simulink model "HIL"  (R2023b)
settings: Solver=VariableStepAuto  StartTime=0.0  StopTime=20.0  RelTol=1e-3
model workspace (MAT data in the model file):
  Iq_ref : Simulink.Parameter (value not decoded)
  Ki_d : Simulink.Parameter (value not decoded)
  Ki_q : Simulink.Parameter (value not decoded)
  Kp_d : Simulink.Parameter (value not decoded)
  Kp_q : Simulink.Parameter (value not decoded)
  P : Simulink.Parameter (value not decoded)
  Torq : Simulink.Parameter (value not decoded)
  Vdc : Simulink.Parameter (value not decoded)
  fe : Simulink.Parameter (value not decoded)
symbols that are objects in the model workspace (value not decoded): fe, Ki_d, Kp_d, P, Torq, Vdc
libraries: instrumentseriallib x3, etargetslib x2, slpidlib x2, mcbcontrolslib x1, dspfdesign x1, dspstat3 x1
(part 2 of 2)

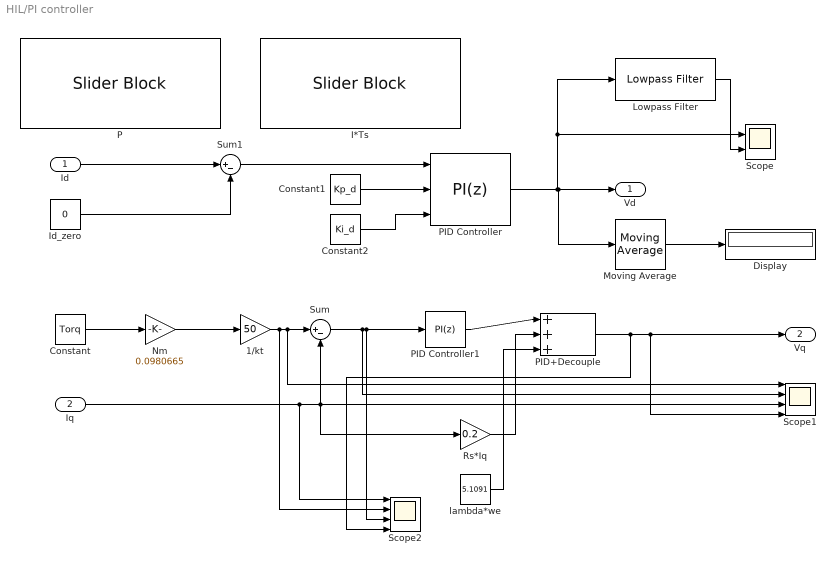
== system HIL/PI controller ==
  Id : Inport
  Iq : Inport  Port=2
  1/kt : Gain  Gain=50
  Constant : Constant  Value=Torq
  Constant1 : Constant  Value=Kp_d
  Constant2 : Constant  Value=Ki_d
  Display : Display
  I*Ts : SliderBlock  ScaleMax=0.1
  Id_zero : Constant  Value=0
  Lowpass Filter : dspfdesign/Lowpass Filter  FilterType=FIR  DesignForMinimumOrder=on  FilterOrder=50  PassbandFrequency=8e3  StopbandFrequency=12e3  PassbandRipple=0.1  StopbandAttenuation=80  SampleRateMode=Specify on dialog  SampleRate=44100  SimulateUsing=Interpreted execution  roundingMode=Floor  coeffsDataTypeStr=fixdt(1,16)
  Moving Average : dspstat3/Moving Average  Method=Sliding window  ForgettingFactorPort=off  SpecifyWindowLength=on  WindowLength=5  OverlapLength=3  AllowArbitraryInputLength=on  ForgettingFactor=0.9  SimulateUsing=Code generation
  Nm : Gain  Gain=0.0980665
  P : SliderBlock  ScaleMin=1.116  ScaleMax=1.12
  PID Controller : slpidlib/PID Controller  Controller=PI  Form=Parallel  TimeDomain=Discrete-time  UseExternalTs=off  SampleTime=1e-3  IntegratorMethod=Forward Euler  FilterMethod=Forward Euler  ControllerParametersSource=external  P=1.13  I=1.885  UseKiTs=on  D=0  N=100  UseFilter=on  TunerSelectOption=Transfer Function Based (PID Tuner App)  ZeroCross=off  InitialConditionSource=internal  InitialConditionForIntegrator=0  InitialConditionForFilter=0  DifferentiatorICPrevScaledInput=0  ExternalReset=none  TrackingMode=off  Kt=1  LimitOutput=on  SatLimitsSource=internal  UpperSaturationLimit=13.8564064606  LowerSaturationLimit=-13.8564064606  LinearizeAsGain=on  AntiWindupMode=back-calculation  Kb=0.8849  LimitIntegrator=off  UpperIntegratorSaturationLimit=inf  LowerIntegratorSaturationLimit=-inf  POutMin=[]  POutMax=[]  IOutMin=[]  IOutMax=[]  DOutMin=[]  DOutMax=[]  NOutMin=[]  NOutMax=[]  SumOutMin=[]  SumOutMax=[]  SaturationOutMin=[]  SaturationOutMax=[]  PParamMin=[]  PParamMax=[]  IParamMin=[]  IParamMax=[]  DParamMin=[]  DParamMax=[]  NParamMin=[]  NParamMax=[]  KbParamMin=[]  KbParamMax=[]  KtParamMin=[]  KtParamMax=[]  KbOutMin=[]  KbOutMax=[]  KtOutMin=[]  KtOutMax=[]  IntegratorOutMin=[]  IntegratorOutMax=[]  FilterOutMin=[]  FilterOutMax=[]  SumI1OutMin=[]  SumI1OutMax=[]  SumI2OutMin=[]  SumI2OutMax=[]  SumI3OutMin=[]  SumI3OutMax=[]  SumI4OutMin=[]  SumI4OutMax=[]  SumDOutMin=[]  SumDOutMax=[]  DifferentiatorOutMin=[]  DifferentiatorOutMax=[]  FilterDiffOutCoefMin=[]  FilterDiffOutCoefMax=[]  ReciprocalOutMin=[]  ReciprocalOutMax=[]  SumDenOutMin=[]  SumDenOutMax=[]  SumNumOutMin=[]  SumNumOutMax=[]  DivideOutMin=[]  DivideOutMax=[]  UdiffTsProdOutMin=[]  UdiffTsProdOutMax=[]  NTsProdOutMin=[]  NTsProdOutMax=[]  UintegralTsProdOutMin=[]  UintegralTsProdOutMax=[]  UngainTsProdOutMin=[]  UngainTsProdOutMax=[]  ClampingZeroOutDataTypeStr=Inherit: Inherit via back propagation  ClampingZeroOutMin=[]  ClampingZeroOutMax=[]  FilterDenConstantOutDataTypeStr=Inherit: Inherit via back propagation  FilterDenConstantOutMin=[]  FilterDenConstantOutMax=[]  PCopyOutDataTypeStr=Inherit: Inherit via back propagation  PCopyOutMin=[]  PCopyOutMax=[]  NCopyOutDataTypeStr=Inherit: Inherit via back propagation  NCopyOutMin=[]  NCopyOutMax=[]  IntegratorContinuousStateAttributes=''  IntegratorStateMustResolveToSignalObject=off  IntegratorRTWStateStorageClass=Auto  FilterContinuousStateAttributes=''  FilterStateMustResolveToSignalObject=off  FilterRTWStateStorageClass=Auto  ParallelPVariant=ExternalParameters  IdealPVariant=Disabled  IVariant=ExternalParameters  DVariant=Disabled  IntegratorVariant=Discrete  SatVariant=Enabled  AWVariant=BackCalculation  PCopyVariant=Disabled  TRVariant=Disabled  FdbkBlocksVariant=Forward  IdealPFdbkVariant=Disabled  SatFdbkVariant=Disabled  DerivativeFilterVariant=Disabled  NVariant=Disabled  NCopyVariant=Disabled_SignalSpec  FilterICVariant=Disabled  IntegratorICVariant=InternalICs  ExternalResetVariant=Disabled  TRSumVariant=Passthrough  SumFdbkVariant=Disabled  SumVariant=Sum_PI  TsampFilterVariant=InternalTs  TsampNgainVariant=Passthrough  TsampIntegralVariant=Disabled_SignalSpec  ExternalSaturationOutDataTypeStr=Inherit: Same as second input
  PID Controller1 : slpidlib/PID Controller  Controller=PI  Form=Parallel  TimeDomain=Discrete-time  UseExternalTs=off  SampleTime=1e-3  IntegratorMethod=Forward Euler  FilterMethod=Forward Euler  ControllerParametersSource=internal  P=1.13  I=1.885  UseKiTs=on  D=0  N=100  UseFilter=on  TunerSelectOption=Transfer Function Based (PID Tuner App)  ZeroCross=off  InitialConditionSource=internal  InitialConditionForIntegrator=0  InitialConditionForFilter=0  DifferentiatorICPrevScaledInput=0  ExternalReset=none  TrackingMode=off  Kt=1  LimitOutput=on  SatLimitsSource=internal  UpperSaturationLimit=13.8564064606  LowerSaturationLimit=-13.8564064606  LinearizeAsGain=on  AntiWindupMode=back-calculation  Kb=0.8849  LimitIntegrator=off  UpperIntegratorSaturationLimit=inf  LowerIntegratorSaturationLimit=-inf  POutMin=[]  POutMax=[]  IOutMin=[]  IOutMax=[]  DOutMin=[]  DOutMax=[]  NOutMin=[]  NOutMax=[]  SumOutMin=[]  SumOutMax=[]  SaturationOutMin=[]  SaturationOutMax=[]  PParamMin=[]  PParamMax=[]  IParamMin=[]  IParamMax=[]  DParamMin=[]  DParamMax=[]  NParamMin=[]  NParamMax=[]  KbParamMin=[]  KbParamMax=[]  KtParamMin=[]  KtParamMax=[]  KbOutMin=[]  KbOutMax=[]  KtOutMin=[]  KtOutMax=[]  IntegratorOutMin=[]  IntegratorOutMax=[]  FilterOutMin=[]  FilterOutMax=[]  SumI1OutMin=[]  SumI1OutMax=[]  SumI2OutMin=[]  SumI2OutMax=[]  SumI3OutMin=[]  SumI3OutMax=[]  SumI4OutMin=[]  SumI4OutMax=[]  SumDOutMin=[]  SumDOutMax=[]  DifferentiatorOutMin=[]  DifferentiatorOutMax=[]  FilterDiffOutCoefMin=[]  FilterDiffOutCoefMax=[]  ReciprocalOutMin=[]  ReciprocalOutMax=[]  SumDenOutMin=[]  SumDenOutMax=[]  SumNumOutMin=[]  SumNumOutMax=[]  DivideOutMin=[]  DivideOutMax=[]  UdiffTsProdOutMin=[]  UdiffTsProdOutMax=[]  NTsProdOutMin=[]  NTsProdOutMax=[]  UintegralTsProdOutMin=[]  UintegralTsProdOutMax=[]  UngainTsProdOutMin=[]  UngainTsProdOutMax=[]  ClampingZeroOutDataTypeStr=Inherit: Inherit via back propagation  ClampingZeroOutMin=[]  ClampingZeroOutMax=[]  FilterDenConstantOutDataTypeStr=Inherit: Inherit via back propagation  FilterDenConstantOutMin=[]  FilterDenConstantOutMax=[]  PCopyOutDataTypeStr=Inherit: Inherit via back propagation  PCopyOutMin=[]  PCopyOutMax=[]  NCopyOutDataTypeStr=Inherit: Inherit via back propagation  NCopyOutMin=[]  NCopyOutMax=[]  IntegratorContinuousStateAttributes=''  IntegratorStateMustResolveToSignalObject=off  IntegratorRTWStateStorageClass=Auto  FilterContinuousStateAttributes=''  FilterStateMustResolveToSignalObject=off  FilterRTWStateStorageClass=Auto  ParallelPVariant=InternalParameters  IdealPVariant=Disabled  IVariant=InternalParameters  DVariant=Disabled  IntegratorVariant=Discrete  SatVariant=Enabled  AWVariant=BackCalculation  PCopyVariant=Disabled  TRVariant=Disabled  FdbkBlocksVariant=Forward  IdealPFdbkVariant=Disabled  SatFdbkVariant=Disabled  DerivativeFilterVariant=Disabled  NVariant=Disabled  NCopyVariant=Disabled_SignalSpec  FilterICVariant=Disabled  IntegratorICVariant=InternalICs  ExternalResetVariant=Disabled  TRSumVariant=Passthrough  SumFdbkVariant=Disabled  SumVariant=Sum_PI  TsampFilterVariant=InternalTs  TsampNgainVariant=Passthrough  TsampIntegralVariant=Disabled_SignalSpec  ExternalSaturationOutDataTypeStr=Inherit: Same as second input
  PID+Decouple : Sum  Inputs=|+++
  Rs*Iq : Gain  Gain=0.2
  Scope : Scope  NumInputPorts=2
  Scope1 : Scope  NumInputPorts=4
  Scope2 : Scope  NumInputPorts=4
  Sum : Sum  Inputs=|+-
  Sum1 : Sum  Inputs=|+-
  lambda*we : Constant  Value=5.1091
  Vd : Outport
  Vq : Outport  Port=2
  wires:
  Iq/1 -> Scope2/1, Rs*Iq/1, Sum/2, Scope1/3
  1/kt/1 -> Scope2/2, Scope1/1, Sum/1
  Id/1 -> Sum1/1
  Id_zero/1 -> Sum1/2
  Sum1/1 -> PID Controller/1
  Sum/1 -> Scope1/2, PID Controller1/1, Scope2/3
  PID Controller/1 -> Lowpass Filter/1, Scope/1, Moving Average/1, Vd/1
  Nm/1 -> 1/kt/1
  Constant/1 -> Nm/1
  Constant1/1 -> PID Controller/2
  Constant2/1 -> PID Controller/3
  Lowpass Filter/1 -> Scope/2
  Moving Average/1 -> Display/1
  Rs*Iq/1 -> PID+Decouple/2
  lambda*we/1 -> PID+Decouple/3
  PID+Decouple/1 -> Scope2/4, Vq/1, Scope1/4
  PID Controller1/1 -> PID+Decouple/1

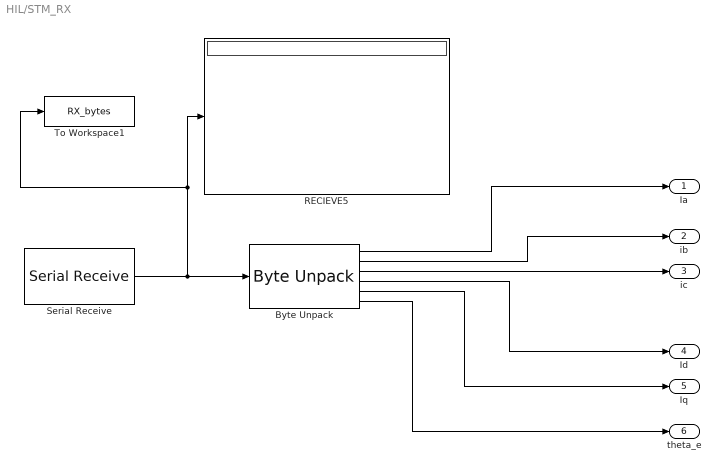
== system HIL/STM_RX ==
  Byte Unpack : etargetslib/Byte Unpack  dimensions={[1 1],[1 1],[1 1],[1 1],[1 1],[1 1]}  datatypes={'single','single','single','single','single','single'}  byteAlign=1
      settings: LibrarySourceBlock=embeddedtargetslib/Host Communication/Byte Unpack
  RECIEVE5 : Display
  Serial Receive : instrumentseriallib/Serial Receive  Priority=1  PortSel=COM11  Port=COM11  ComPort=COM11  DataType=uint8  SaveDataType=uint8  ToggleHeader=on  Header=[170]  ToggleTerminator=on  Terminator=Custom terminator  CustomTerminator=[85]  InputFormat=Column major  ToggleDataSize=on  DataSize=[24 1]  EnableBlockingMode=on  ActionDataUnavailable=Output last received value  ActionWhenDataUnavailable=Output last received value  CustomValue=0  SampleTime=-1  SimulateUsing=Interpreted execution  BlockInModel=on  aMode=1
      settings: LibrarySourceBlock=embeddedtargetslib/Host Communication/Serial Receive
  To Workspace1 : ToWorkspace  VariableName=RX_bytes  SampleTime=-1
  Ia : Outport
  ib : Outport  Port=2
  ic : Outport  Port=3
  Id : Outport  Port=4
  Iq : Outport  Port=5
  theta_e : Outport  Port=6
  wires:
  Byte Unpack/3 -> ic/1
  Serial Receive/1 -> To Workspace1/1, RECIEVE5/1, Byte Unpack/1
  Byte Unpack/1 -> Ia/1
  Byte Unpack/2 -> ib/1
  Byte Unpack/4 -> Id/1
  Byte Unpack/5 -> Iq/1
  Byte Unpack/6 -> theta_e/1

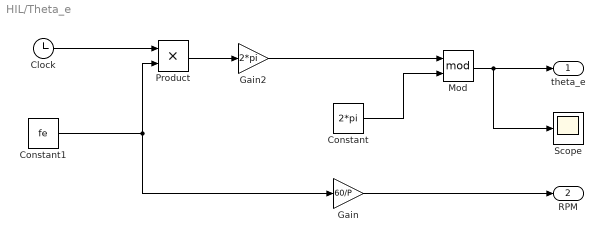
== system HIL/Theta_e ==
  Clock : Clock
  Constant : Constant  Value=2*pi  SampleTime=1e-3
  Constant1 : Constant  Value=fe  SampleTime=1e-3
  Gain : Gain  Gain=60/P
  Gain2 : Gain  Gain=2*pi
  Mod : Math  Operator=mod
  Product : Product
  Scope : Scope
  theta_e : Outport  OutDataTypeStr=double  SampleTime=1e-3
  RPM : Outport  Port=2
  wires:
  Gain2/1 -> Mod/1
  Constant/1 -> Mod/2
  Mod/1 -> Scope/1, theta_e/1
  Gain/1 -> RPM/1
  Product/1 -> Gain2/1
  Constant1/1 -> Product/2, Gain/1
  Clock/1 -> Product/1

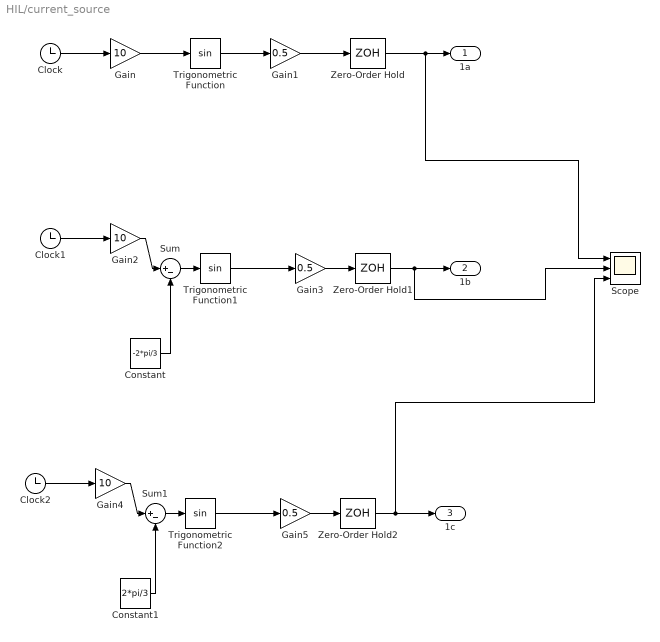
== system HIL/current_source ==
  Clock : Clock
  Clock1 : Clock
  Clock2 : Clock
  Constant : Constant  Value=-2*pi/3
  Constant1 : Constant  Value=2*pi/3
  Gain : Gain  Gain=10
  Gain1 : Gain  Gain=0.5
  Gain2 : Gain  Gain=10
  Gain3 : Gain  Gain=0.5
  Gain4 : Gain  Gain=10
  Gain5 : Gain  Gain=0.5
  Scope : Scope  NumInputPorts=3
  Sum : Sum  Inputs=|+-
  Sum1 : Sum  Inputs=|+-
  Trigonometric Function : Trigonometry
  Trigonometric Function1 : Trigonometry
  Trigonometric Function2 : Trigonometry
  Zero-Order Hold : ZeroOrderHold  SampleTime=1e-3
  Zero-Order Hold1 : ZeroOrderHold  SampleTime=1e-3
  Zero-Order Hold2 : ZeroOrderHold  SampleTime=1e-3
  1a : Outport
  1b : Outport  Port=2
  1c : Outport  Port=3
  wires:
  Clock/1 -> Gain/1
  Gain/1 -> Trigonometric Function/1
  Trigonometric Function/1 -> Gain1/1
  Zero-Order Hold/1 -> Scope/1, 1a/1
  Gain1/1 -> Zero-Order Hold/1
  Gain3/1 -> Zero-Order Hold1/1
  Clock1/1 -> Gain2/1
  Zero-Order Hold1/1 -> Scope/2, 1b/1
  Trigonometric Function1/1 -> Gain3/1
  Gain2/1 -> Sum/1
  Constant/1 -> Sum/2
  Sum/1 -> Trigonometric Function1/1
  Gain4/1 -> Sum1/1
  Sum1/1 -> Trigonometric Function2/1
  Gain5/1 -> Zero-Order Hold2/1
  Trigonometric Function2/1 -> Gain5/1
  Clock2/1 -> Gain4/1
  Zero-Order Hold2/1 -> Scope/3, 1c/1
  Constant1/1 -> Sum1/2
